simulink model "main"  (R2022a)
settings: Solver=ode3  StartTime=0.0  StopTime=10.0  RelTol=1e-3  EnableMultiTasking=on
model workspace (MAT data in the model file):
  BER = 1e-09
  Br = 1000000000
  Dr = 0.01
  Dt = 0.01
  F = 6
  G = 200
  GT = 0.012
  Ib = 5e-10
  Id = 1e-09
  Is = 5e-09
  Keff = 0.01
  Lil = -2
  Lin = -1.5
  Lout = -1.5
  M = 4
  Mer = 12
  Pavg = 0.0065
  Pback = 1e-13
  Pmax = 0.012
  Pmin = 0.001
  RIN = -145
  Rl = 100
  Tr = 300
  d = 1000
  d_gamma = 1e-09
  ja = 1e-05
  k = 2
  lambda = 8.5e-07
  n = 0.59
  nr = 0.8
  nsp = 2
  nt = 0.8
  u = 1
settings Model: Creator=keged  LastModifiedBy=keged
settings SolverCC: AutoInsertRateTranBlk=on
settings DataIOCC: SaveOutput=off  SaveTime=off
settings OptimizationCC: DefaultParameterBehavior=Inlined  InlineInvariantSignals=on  EnhancedBackFolding=on  PassReuseOutputArgsAs=Individual arguments  StateBitsets=on  DataBitsets=on  ZeroExternalMemoryAtStartup=off  ZeroInternalMemoryAtStartup=off  NoFixptDivByZeroProtection=on  LifeSpan=1  OptimizeBlockOrder=speed  DifferentSizesBufferReuse=on  EfficientTunableParamExpr=on
settings DebuggingCC: ParameterTunabilityLossMsg=error
settings HardwareCC: ProdBitPerPointer=32  ProdBitPerSizeT=32  ProdBitPerPtrDiffT=32  ProdLargestAtomicFloat=None  ProdIntDivRoundTo=Floor  ProdWordSize=32  ProdHWDeviceType=Generic->Custom
settings SFSimCC: MATLABDynamicMemAlloc=off
settings RTWCC: SystemTargetFile=ert.tlc  TLCOptions=-p0  GenCodeOnly=on  TemplateMakefile=ert_default_tmf  GenerateReport=on  RTWVerbose=off  IncludeHyperlinkInReport=on  LaunchReport=on
settings CodeAppCC: ForceParamTrailComments=on  IgnoreCustomStorageClasses=off  OperatorAnnotations=on  SimulinkDataObjDesc=on  SFDataObjDesc=on  CustomSymbolStrGlobalVar=rt$N$M  CustomSymbolStrType=$N$M  CustomSymbolStrFcn=$N$M$F  CustomSymbolStrMacro=$N$M  InsertBlockDesc=on
settings ERTTargetCC: TargetLangStandard=C99 (ISO)  CodeReplacementLibrary=ISO_C  GenerateSampleERTMain=on  IncludeMdlTerminateFcn=off  SuppressErrorStatus=on  SupportAbsoluteTime=off  PurelyIntegerCode=on  SupportNonFinite=off  SupportComplex=off  InlinedParameterPlacement=NonHierarchical  RootIOFormat=Structure reference  ERTCustomFileTemplate=example_file_process.tlc

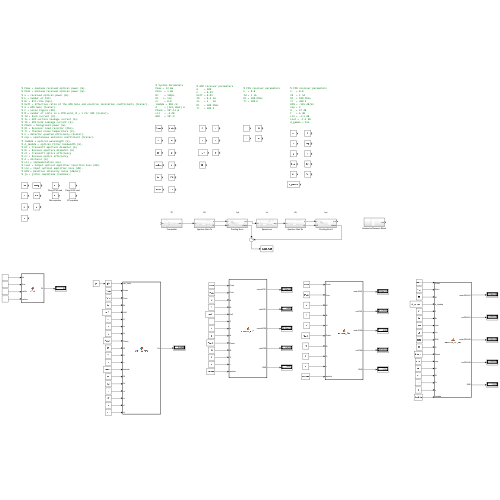
[thumbnail: Simulink's stored preview of the top-level diagram]
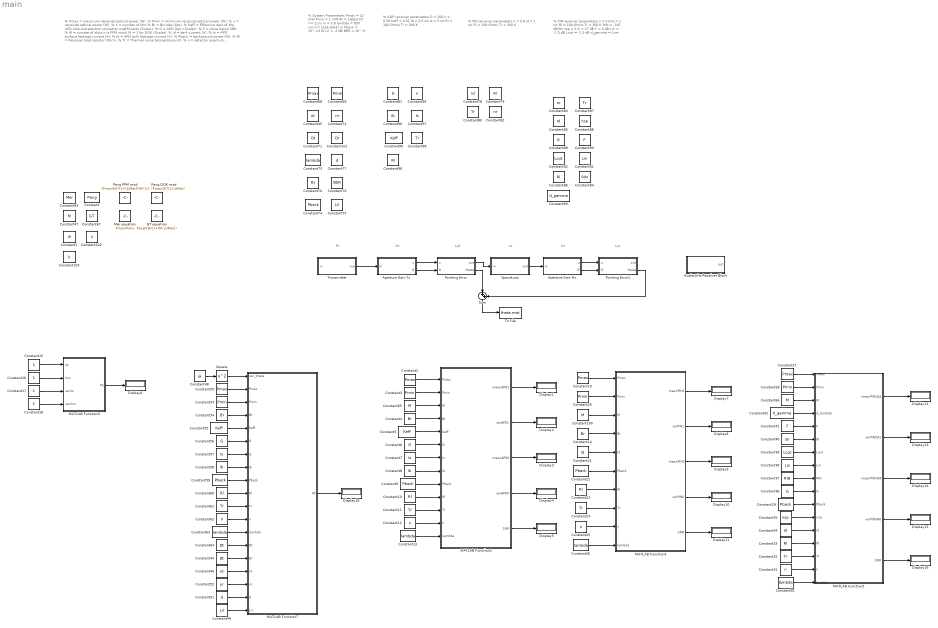
== system main ==
  note: Pt
  note: % PIN receiver parameters
      | n = 0.8
      | Id = 1 nA
      | Rl = 100 Ohms
      | Tr = 300 K
  note: % Pmax = maximum received optical power (W).
      | % Pmin = minimum received optical power (W).
      | % u = received optical power (W).
      | % k = number of bits
      | % Br = Bit rate (bps).
      | % Keff = Effective ratio of the APD hole and electron ionization coefficients (Scalar).
      | % G = APD Gain (Scalar).
      | % F = noise figure (dB).
      | % M = number of slots in a PPM word, M = 1 for OOK (Scalar).
      | % Id = dark current (A).
      | % Is = APD surface leakage current (A).
      | % Ib = APD bulk leakage current (A).
      | % Pback = background power (W).
      | % Rl = Receiver load resistor (Ohm).
      | % Tr = Thermal noise temperature (K).
      | % n = detector quantum efficiency (Scalar).
      | % nsp = spontaneous emission coefficient (Scalar).
      | % lambda = optical wavelength (m).
      | % d_lambda = optical filter bandwidth (m).
      | % Dt = Transmitt aperture diameter (m)
      | % Dr = Recieve aperture diameter (m)
      | % nt = Transmitt optics efficiency
      | % nr = Recieve optics efficiency
      | % d = distance (m)
      | % Lil = implementation loss
      | % Lout = Output optical amplifier insertion loss (dB).
      | % Lin = Input optical amplifier loss (dB).
      | % RIN = Relative intensity noise (dB/Hz).
      | % ja = jitter amplitude (radians).
  note: % ADP receiver parameters
      | G = 200
      | n = 0.59
      | Keff = 0.01
      | Ib = 0.5 nA
      | Is = 5 nA
      | Rl = 100 Ohms
      | Tr = 300 K
  note: % PIN receiver parameters
      | n = 0.8
      | Id = 1 nA
      | Rl = 100 Ohms
      | Tr = 300 K
      | RIN = -145 dB/Hz
      | nsp = 2
      | G = 27 dB
      | F = 6 dB
      | Lin = -1.5 dB
      | Lout = -1.5 dB
      | d_gamma = 1nm
  note: % System Parameters
      | Pmax = 12 mW
      | Pmin = 1 mW
      | Br = 1Gbps
      | Dt <= 1cm
      | nr = 0.8
      | lambda = 850 cm
      | d = [1e3,10e3] m
      | Pback = 10^-13 W
      | Lil = -2 dB
      | BER = 10^-9
  note: Gt
  note: Lpt
  note: Ls
  note: Lpr
  note: Gr
  Aperture Gain Rx : Subsystem
  Aperture Gain Tx : Subsystem
  Avalanche Receiver Block : Subsystem
  Constant : Constant  Value=Pavg
  Constant1 : Constant  Value=ja
  Constant{10,23,33,60,79,86,98} (7 alike) : Constant  Value=Rl
  Constant{47,65..66,100} (4 alike) : Constant  Value=M
  Constant101 : Constant  Value=Dr
  Constant102 : Constant  Value=u
  Constant103 : Constant  Value=k
  Constant{11,24,32,61,80,87,99} (7 alike) : Constant  Value=Tr
  Constant{12,25,31,62,94} (5 alike) : Constant  Value=n
  Constant{13,26,30,63,73} (5 alike) : Constant  Value=lambda
  Constant{4,14,40,54,70} (5 alike) : Constant  Value=Br
  Constant{15..18} (4 alike) : Constant
  Constant{2,19,27,50,68} (5 alike) : Constant  Value=Pmax
  Constant{3,20,28,53,69} (5 alike) : Constant  Value=Pmin
  Constant{21,34,78,85} (4 alike) : Constant  Value=Id
  Constant{9,22,29,59,74} (5 alike) : Constant  Value=Pback
  Constant35 : Constant  Value=nsp
  Constant{6,36,56,81,89} (5 alike) : Constant  Value=G
  Constant37 : Constant  Value=RIN
  Constant38 : Constant  Value=Lin
  Constant39 : Constant  Value=Lout
  Constant41 : Constant  Value=F
  Constant42 : Constant  Value=d_gamma
  Constant43 : Constant  Value=Mer
  Constant44 : Constant  Value=Dt
  Constant45 : Constant  Value=nt
  Constant46 : Constant  Value=nt
  Constant48 : Constant  Value=ja
  Constant49 : Constant  Value=Lil
  Constant5 : Constant  Value=Keff
  Constant51 : Constant  Value=d
  Constant{52,72,82..83} (4 alike) : Constant  Value=nr
  Constant55 : Constant  Value=Keff
  Constant57 : Constant  Value=Is
  Constant58 : Constant  Value=Ib
  Constant64 : Constant  Value=Dt
  Constant67 : Constant  Value=GT
  Constant7 : Constant  Value=Is
  Constant71 : Constant  Value=Dt
  Constant75 : Constant  Value=Lil
  Constant76 : Constant  Value=BER
  Constant77 : Constant  Value=d
  Constant8 : Constant  Value=Ib
  Constant84 : Constant  Value=RIN
  Constant88 : Constant  Value=nsp
  Constant90 : Constant  Value=F
  Constant91 : Constant  Value=Lin
  Constant92 : Constant  Value=Lout
  Constant93 : Constant  Value=d_gamma
  Constant95 : Constant  Value=Keff
  Constant96 : Constant  Value=Ib
  Constant97 : Constant  Value=Is
  Display{1..16,18} (17 alike) : Display
  GT equation : Constant  Value=Pavg*(M/(1+(M-1)/Mer))
  MATLAB Function2 : MATLAB Function  TreatAsAtomicUnit=on  RTWFcnName=Pointing
      settings: RTWFcnNameOpts=Use subsystem name  RTWFileNameOpts=Use subsystem name
  MATLAB Function3 : MATLAB Function  TreatAsAtomicUnit=on  RTWFcnName=Pointing
      settings: RTWFcnNameOpts=Use subsystem name  RTWFileNameOpts=Use subsystem name
  MATLAB Function4 : MATLAB Function  TreatAsAtomicUnit=on  RTWFcnName=Pointing
      settings: RTWFcnNameOpts=Use subsystem name  RTWFileNameOpts=Use subsystem name
  MATLAB Function5 : MATLAB Function  TreatAsAtomicUnit=on  RTWFcnName=Pointing
      settings: RTWFcnNameOpts=Use subsystem name  RTWFileNameOpts=Use subsystem name
  MATLAB Function7 : MATLAB Function  TreatAsAtomicUnit=on  RTWFcnName=Pointing
      settings: RTWFcnNameOpts=Use subsystem name  RTWFileNameOpts=Use subsystem name
  Mer equation : Constant  Value=Pmax/Pmin
  Pavg OOK mod : Constant  Value=(Pmax/2)*(1+1/Mer)
  Pavg PPM mod : Constant  Value=(Pmax/M)*(1+(1/Mer)*(M-1))
  Pointing Error : Subsystem
  Pointing Error1 : Subsystem
  SpaceLoss : Subsystem
  Square : Math  Operator=square
  Sum : Sum  Inputs=|++
  To File : ToFile  Filename=theta.mat  SaveFormat=Timeseries
  Transmitter : Subsystem
  wires:
  MATLAB Function2/1(meanAPD1) -> Display1/1
  Constant3/1 -> MATLAB Function2/2(Pmin)
  Constant2/1 -> MATLAB Function2/1(Pmax)
  Constant65/1 -> MATLAB Function2/3(M)
  Constant4/1 -> MATLAB Function2/4(Br)
  Constant5/1 -> MATLAB Function2/5(Keff)
  Constant6/1 -> MATLAB Function2/6(G)
  Constant7/1 -> MATLAB Function2/7(Is)
  Constant8/1 -> MATLAB Function2/8(Ib)
  Constant9/1 -> MATLAB Function2/9(Pback)
  Constant10/1 -> MATLAB Function2/10(Rl)
  Constant11/1 -> MATLAB Function2/11(Tr)
  Constant12/1 -> MATLAB Function2/12(n)
  Constant13/1 -> MATLAB Function2/13(lambda)
  MATLAB Function2/2(varAPD1) -> Display2/1
  MATLAB Function2/3(meanAPD0) -> Display3/1
  MATLAB Function2/4(varAPD0) -> Display4/1
  MATLAB Function2/5(SNR) -> Display5/1
  MATLAB Function3/1(Pb) -> Display6/1
  Constant16/1 -> MATLAB Function3/2(Xns)
  Constant15/1 -> MATLAB Function3/1(Xs)
  Constant17/1 -> MATLAB Function3/3(varXs)
  Constant18/1 -> MATLAB Function3/4(varXns)
  MATLAB Function4/4(varPIN0) -> Display10/1
  MATLAB Function4/5(SNR) -> Display11/1
  Constant100/1 -> MATLAB Function4/3(M)
  Constant24/1 -> MATLAB Function4/8(Tr)
  Constant22/1 -> MATLAB Function4/6(Pback)
  MATLAB Function4/2(varPIN1) -> Display8/1
  Constant21/1 -> MATLAB Function4/5(Id)
  MATLAB Function4/3(meanPIN0) -> Display9/1
  Constant23/1 -> MATLAB Function4/7(Rl)
  MATLAB Function4/1(meanPIN1) -> Display7/1
  Constant25/1 -> MATLAB Function4/9(n)
  Constant14/1 -> MATLAB Function4/4(Br)
  Constant20/1 -> MATLAB Function4/2(Pmin)
  Constant26/1 -> MATLAB Function4/10(lambda)
  Constant19/1 -> MATLAB Function4/1(Pmax)
  MATLAB Function5/4(varPINOA0) -> Display15/1
  MATLAB Function5/5(SNR) -> Display16/1
  Constant41/1 -> MATLAB Function5/5(F)
  Constant66/1 -> MATLAB Function5/3(M)
  Constant39/1 -> MATLAB Function5/7(Lout)
  Constant32/1 -> MATLAB Function5/15(Tr)
  Constant29/1 -> MATLAB Function5/11(Pback)
  MATLAB Function5/2(varPINOA1) -> Display13/1
  Constant36/1 -> MATLAB Function5/10(G)
  Constant42/1 -> MATLAB Function5/4(d_lambda)
  MATLAB Function5/3(meanPINOA0) -> Display14/1
  Constant33/1 -> MATLAB Function5/14(Rl)
  MATLAB Function5/1(meanPINOA1) -> Display12/1
  Constant31/1 -> MATLAB Function5/16(n)
  Constant40/1 -> MATLAB Function5/6(Br)
  Constant28/1 -> MATLAB Function5/2(Pmin)
  Constant30/1 -> MATLAB Function5/17(lambda)
  Constant27/1 -> MATLAB Function5/1(Pmax)
  Constant34/1 -> MATLAB Function5/13(Id)
  Constant35/1 -> MATLAB Function5/12(nsp)
  Constant37/1 -> MATLAB Function5/9(RIN)
  Constant38/1 -> MATLAB Function5/8(Lin)
  MATLAB Function7/1(Pb) -> Display18/1
  Square/1 -> MATLAB Function7/1(var_theta)
  Constant50/1 -> MATLAB Function7/2(Pmax)
  Constant53/1 -> MATLAB Function7/3(Pmin)
  Constant54/1 -> MATLAB Function7/4(Br)
  Constant55/1 -> MATLAB Function7/5(Keff)
  Constant56/1 -> MATLAB Function7/6(G)
  Constant57/1 -> MATLAB Function7/7(Is)
  Constant58/1 -> MATLAB Function7/8(Ib)
  Constant59/1 -> MATLAB Function7/9(Pback)
  Constant60/1 -> MATLAB Function7/10(Rl)
  Constant61/1 -> MATLAB Function7/11(Tr)
  Constant62/1 -> MATLAB Function7/12(n)
  Constant63/1 -> MATLAB Function7/13(lambda)
  Constant64/1 -> MATLAB Function7/14(Dt)
  Constant44/1 -> MATLAB Function7/15(Dr)
  Constant46/1 -> MATLAB Function7/16(nt)
  Constant52/1 -> MATLAB Function7/17(nr)
  Constant51/1 -> MATLAB Function7/18(d)
  Constant49/1 -> MATLAB Function7/19(Lil)
  Transmitter/1(out) -> Aperture Gain Tx/1(in)
  Aperture Gain Tx/1(u) -> Pointing Error/1(u)
  Aperture Gain Tx/2(G) -> Pointing Error/2(G)
  Constant48/1 -> Square/1
  Pointing Error/1(out) -> SpaceLoss/1(in)
  SpaceLoss/1(out) -> Aperture Gain Rx/1(in)
  Pointing Error/2(theta) -> Sum/1
  Sum/1 -> To File/1
  Aperture Gain Rx/1(u) -> Pointing Error1/1(u)
  Aperture Gain Rx/2(G) -> Pointing Error1/2(G)
  Pointing Error1/2(theta) -> Sum/2

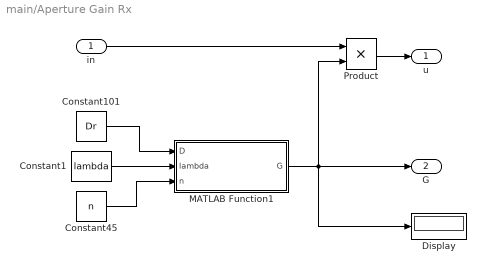
== system main/Aperture Gain Rx ==
  in : Inport
  Constant1 : Constant  Value=lambda
  Constant101 : Constant  Value=Dr
  Constant45 : Constant  Value=n
  Display : Display
  MATLAB Function1 : MATLAB Function  TreatAsAtomicUnit=on  RTWFcnName=Pointing
      settings: RTWFcnNameOpts=Use subsystem name  RTWFileNameOpts=Use subsystem name
  Product : Product
  u : Outport
  G : Outport  Port=2
  wires:
  Constant101/1 -> MATLAB Function1/1(D)
  Constant45/1 -> MATLAB Function1/3(n)
  Constant1/1 -> MATLAB Function1/2(lambda)
  MATLAB Function1/1(G) -> Display/1, Product/2, G/1
  Product/1 -> u/1
  in/1 -> Product/1

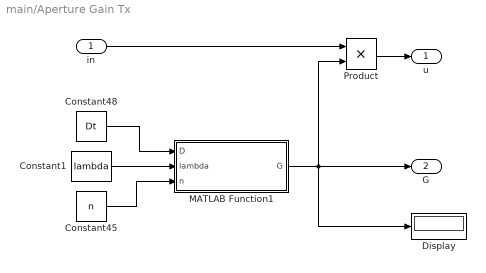
== system main/Aperture Gain Tx ==
  in : Inport
  Constant1 : Constant  Value=lambda
  Constant45 : Constant  Value=n
  Constant48 : Constant  Value=Dt
  Display : Display
  MATLAB Function1 : MATLAB Function  TreatAsAtomicUnit=on  RTWFcnName=Pointing
      settings: RTWFcnNameOpts=Use subsystem name  RTWFileNameOpts=Use subsystem name
  Product : Product
  u : Outport
  G : Outport  Port=2
  wires:
  Constant48/1 -> MATLAB Function1/1(D)
  Constant45/1 -> MATLAB Function1/3(n)
  Constant1/1 -> MATLAB Function1/2(lambda)
  MATLAB Function1/1(G) -> Display/1, Product/2, G/1
  Product/1 -> u/1
  in/1 -> Product/1

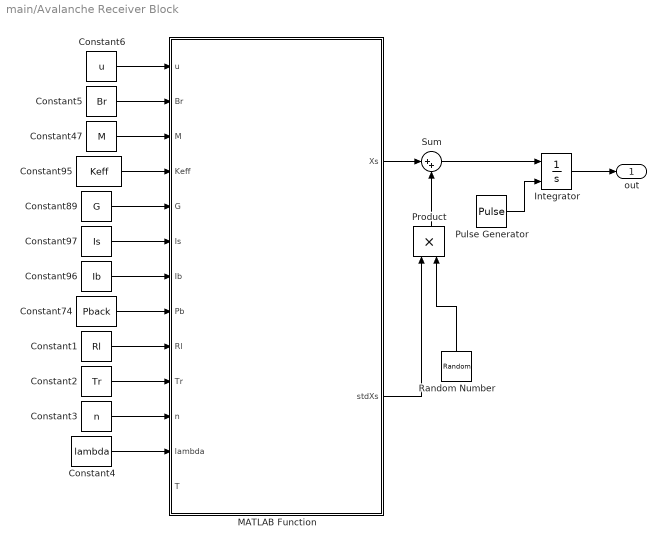
== system main/Avalanche Receiver Block ==
  Constant1 : Constant  Value=Rl
  Constant2 : Constant  Value=Tr
  Constant3 : Constant  Value=n
  Constant4 : Constant  Value=lambda
  Constant47 : Constant  Value=M
  Constant5 : Constant  Value=Br
  Constant6 : Constant  Value=u
  Constant74 : Constant  Value=Pback
  Constant89 : Constant  Value=G
  Constant95 : Constant  Value=Keff
  Constant96 : Constant  Value=Ib
  Constant97 : Constant  Value=Is
  Integrator : Integrator  ExternalReset=rising
  MATLAB Function : MATLAB Function  TreatAsAtomicUnit=on
  Product : Product
  Pulse Generator : DiscretePulseGenerator  PulseType=Time based  Period=k/Br  PulseWidth=k/M/Br
  Random Number : RandomNumber  SampleTime=0.1
  Sum : Sum  Inputs=|++
  out : Outport
  wires:
  Constant47/1 -> MATLAB Function/3(M)
  Constant95/1 -> MATLAB Function/4(Keff)
  Constant89/1 -> MATLAB Function/5(G)
  Constant97/1 -> MATLAB Function/6(Is)
  Constant96/1 -> MATLAB Function/7(Ib)
  Constant1/1 -> MATLAB Function/9(Rl)
  Constant2/1 -> MATLAB Function/10(Tr)
  Constant3/1 -> MATLAB Function/11(n)
  Constant4/1 -> MATLAB Function/12(lambda)
  Constant6/1 -> MATLAB Function/1(u)
  Constant5/1 -> MATLAB Function/2(Br)
  Constant74/1 -> MATLAB Function/8(Pb)
  MATLAB Function/2(stdXs) -> Product/1
  Random Number/1 -> Product/2
  Product/1 -> Sum/2
  MATLAB Function/1(Xs) -> Sum/1
  Integrator/1 -> out/1
  Sum/1 -> Integrator/1
  Pulse Generator/1 -> Integrator/2

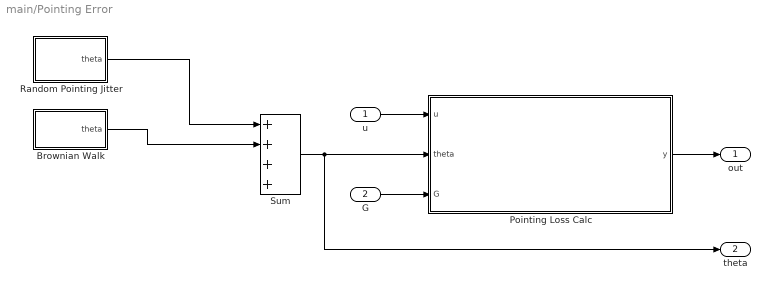
== system main/Pointing Error ==
  u : Inport
  G : Inport  Port=2
  Brownian Walk : Subsystem
  Pointing Loss Calc : Subsystem
  Random Pointing Jitter : Subsystem
  Sum : Sum  Inputs=++++  InputSameDT=on
  out : Outport
  theta : Outport  Port=2
  wires:
  u/1 -> Pointing Loss Calc/1(u)
  Pointing Loss Calc/1(y) -> out/1
  G/1 -> Pointing Loss Calc/3(G)
  Random Pointing Jitter/1(theta) -> Sum/1
  Sum/1 -> Pointing Loss Calc/2(theta), theta/1
  Brownian Walk/1(theta) -> Sum/2

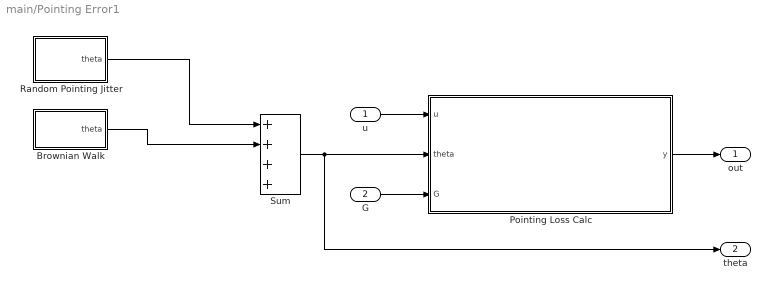
== system main/Pointing Error1 ==
  u : Inport
  G : Inport  Port=2
  Brownian Walk : Subsystem
  Pointing Loss Calc : Subsystem
  Random Pointing Jitter : Subsystem
  Sum : Sum  Inputs=++++  InputSameDT=on
  out : Outport
  theta : Outport  Port=2
  wires:
  u/1 -> Pointing Loss Calc/1(u)
  Pointing Loss Calc/1(y) -> out/1
  G/1 -> Pointing Loss Calc/3(G)
  Random Pointing Jitter/1(theta) -> Sum/1
  Sum/1 -> theta/1, Pointing Loss Calc/2(theta)
  Brownian Walk/1(theta) -> Sum/2

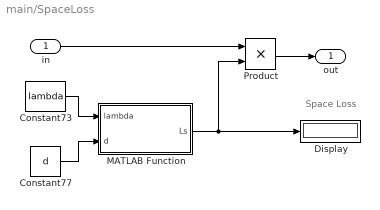
== system main/SpaceLoss ==
  note: Space Loss
  in : Inport
  Constant73 : Constant  Value=lambda
  Constant77 : Constant  Value=d
  Display : Display
  MATLAB Function : MATLAB Function  TreatAsAtomicUnit=on
  Product : Product
  out : Outport
  wires:
  MATLAB Function/1(Ls) -> Display/1, Product/2
  in/1 -> Product/1
  Product/1 -> out/1
  Constant73/1 -> MATLAB Function/1(lambda)
  Constant77/1 -> MATLAB Function/2(d)

== system main/Transmitter ==
  in : Inport
  Constant : Constant
  Constant1 : Constant  Value=1/Mer
  Gain : Gain  Gain=GT
  Switch : Switch  Criteria=u2 > Threshold  SaturateOnIntegerOverflow=off  InputSameDT=off
  out : Outport
  wires:
  in/1 -> Switch/2
  Constant/1 -> Switch/1
  Constant1/1 -> Switch/3
  Gain/1 -> out/1
  Switch/1 -> Gain/1

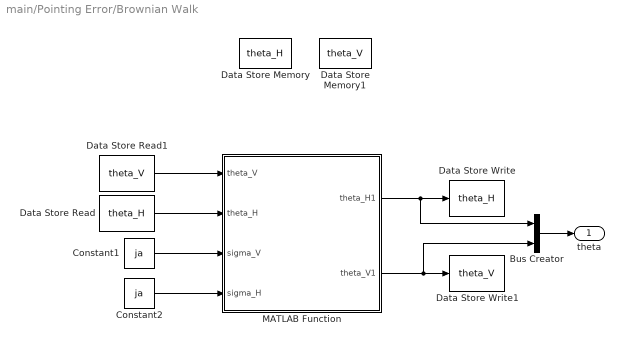
== system main/Pointing Error/Brownian Walk ==
  Bus Creator : BusCreator  Inputs=2
  Constant1 : Constant  Value=ja
  Constant2 : Constant  Value=ja
  Data Store Memory : DataStoreMemory  DataStoreName=theta_H  WriteAfterWriteMsg=warning  ShowAdditionalParam=off
  Data Store Memory1 : DataStoreMemory  DataStoreName=theta_V  WriteAfterWriteMsg=warning  ShowAdditionalParam=off
  Data Store Read : DataStoreRead  DataStoreName=theta_H  IndexOptions=Index vector (dialog)  Indices=1  OutputSizes=1
  Data Store Read1 : DataStoreRead  DataStoreName=theta_V  IndexOptions=Index vector (dialog)  Indices=1  OutputSizes=1
  Data Store Write : DataStoreWrite  DataStoreName=theta_H  IndexOptions=Index vector (dialog)  Indices=1  OutputSizes=1
  Data Store Write1 : DataStoreWrite  DataStoreName=theta_V  IndexOptions=Index vector (dialog)  Indices=1  OutputSizes=1
  MATLAB Function : MATLAB Function  TreatAsAtomicUnit=on
  theta : Outport
  wires:
  MATLAB Function/1(theta_H1) -> Bus Creator/1, Data Store Write/1
  Data Store Read/1 -> MATLAB Function/2(theta_H)
  Data Store Read1/1 -> MATLAB Function/1(theta_V)
  MATLAB Function/2(theta_V1) -> Bus Creator/2, Data Store Write1/1
  Bus Creator/1 -> theta/1
  Constant1/1 -> MATLAB Function/3(sigma_V)
  Constant2/1 -> MATLAB Function/4(sigma_H)

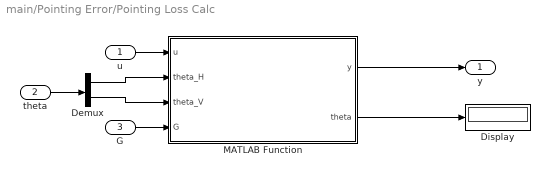
== system main/Pointing Error/Pointing Loss Calc ==
  u : Inport
  theta : Inport  Port=2
  G : Inport  Port=3
  Demux : Demux  Outputs=2
  Display : Display
  MATLAB Function : MATLAB Function  TreatAsAtomicUnit=on
  y : Outport
  wires:
  MATLAB Function/2(theta) -> Display/1
  G/1 -> MATLAB Function/4(G)
  u/1 -> MATLAB Function/1(u)
  MATLAB Function/1(y) -> y/1
  theta/1 -> Demux/1
  Demux/2 -> MATLAB Function/3(theta_V)
  Demux/1 -> MATLAB Function/2(theta_H)

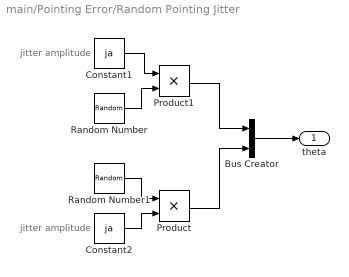
== system main/Pointing Error/Random Pointing Jitter ==
  note: jitter amplitude
  note: jitter amplitude
  Bus Creator : BusCreator  Inputs=2
  Constant1 : Constant  Value=ja
  Constant2 : Constant  Value=ja
  Product : Product
  Product1 : Product
  Random Number : RandomNumber  SampleTime=0.1
  Random Number1 : RandomNumber  SampleTime=0.1
  theta : Outport
  wires:
  Random Number1/1 -> Product/1
  Constant2/1 -> Product/2
  Constant1/1 -> Product1/1
  Random Number/1 -> Product1/2
  Product1/1 -> Bus Creator/1
  Product/1 -> Bus Creator/2
  Bus Creator/1 -> theta/1

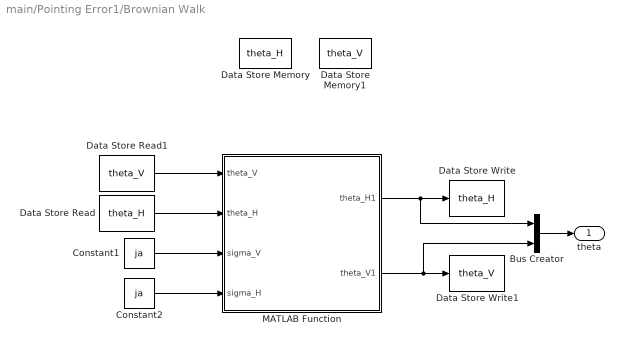
== system main/Pointing Error1/Brownian Walk ==
  Bus Creator : BusCreator  Inputs=2
  Constant1 : Constant  Value=ja
  Constant2 : Constant  Value=ja
  Data Store Memory : DataStoreMemory  DataStoreName=theta_H  WriteAfterWriteMsg=warning  ShowAdditionalParam=off
  Data Store Memory1 : DataStoreMemory  DataStoreName=theta_V  WriteAfterWriteMsg=warning  ShowAdditionalParam=off
  Data Store Read : DataStoreRead  DataStoreName=theta_H  IndexOptions=Index vector (dialog)  Indices=1  OutputSizes=1
  Data Store Read1 : DataStoreRead  DataStoreName=theta_V  IndexOptions=Index vector (dialog)  Indices=1  OutputSizes=1
  Data Store Write : DataStoreWrite  DataStoreName=theta_H  IndexOptions=Index vector (dialog)  Indices=1  OutputSizes=1
  Data Store Write1 : DataStoreWrite  DataStoreName=theta_V  IndexOptions=Index vector (dialog)  Indices=1  OutputSizes=1
  MATLAB Function : MATLAB Function  TreatAsAtomicUnit=on
  theta : Outport
  wires:
  MATLAB Function/1(theta_H1) -> Bus Creator/1, Data Store Write/1
  Data Store Read/1 -> MATLAB Function/2(theta_H)
  Data Store Read1/1 -> MATLAB Function/1(theta_V)
  MATLAB Function/2(theta_V1) -> Bus Creator/2, Data Store Write1/1
  Bus Creator/1 -> theta/1
  Constant1/1 -> MATLAB Function/3(sigma_V)
  Constant2/1 -> MATLAB Function/4(sigma_H)

== system main/Pointing Error1/Pointing Loss Calc ==
  u : Inport
  theta : Inport  Port=2
  G : Inport  Port=3
  Demux : Demux  Outputs=2
  Display : Display
  MATLAB Function : MATLAB Function  TreatAsAtomicUnit=on
  y : Outport
  wires:
  MATLAB Function/2(theta) -> Display/1
  G/1 -> MATLAB Function/4(G)
  u/1 -> MATLAB Function/1(u)
  MATLAB Function/1(y) -> y/1
  theta/1 -> Demux/1
  Demux/1 -> MATLAB Function/2(theta_H)
  Demux/2 -> MATLAB Function/3(theta_V)

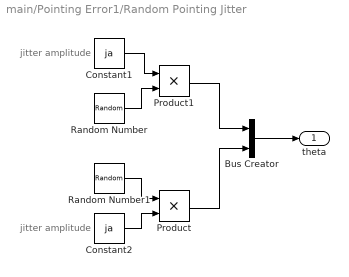
== system main/Pointing Error1/Random Pointing Jitter ==
  note: jitter amplitude
  note: jitter amplitude
  Bus Creator : BusCreator  Inputs=2
  Constant1 : Constant  Value=ja
  Constant2 : Constant  Value=ja
  Product : Product
  Product1 : Product
  Random Number : RandomNumber  SampleTime=0.1
  Random Number1 : RandomNumber  SampleTime=0.1
  theta : Outport
  wires:
  Random Number1/1 -> Product/1
  Constant2/1 -> Product/2
  Constant1/1 -> Product1/1
  Random Number/1 -> Product1/2
  Product1/1 -> Bus Creator/1
  Product/1 -> Bus Creator/2
  Bus Creator/1 -> theta/1

== matlab function main/Pointing Error/Brownian Walk/MATLAB Function ==
  data: theta_V input; theta_H1 output; theta_H input; sigma_V input; sigma_H input; theta_V1 output
function [theta_H1, theta_V1] = brownian_vib(theta_V, theta_H, sigma_V, sigma_H)

%Generates a stochastic random walking motion.
%Sets the standard deviation of the step size for the brownian walk.
d_sigma_H = sigma_H/100;

%Generates a step of random length and direction along the azimuthal axis.
d_theta_H = randn()*d_sigma_H - theta_H*d_sigma_H/sigma_H;

%the new error angle is produced by adding the random step the the current
%error angle.
theta_H1 = theta_H + d_theta_H;

%The same principle for the elevation axis.
d_sigma_V = sigma_V/100;
d_theta_V = randn()*d_sigma_V - theta_V*d_sigma_V/sigma_V;

theta_V1 = theta_V + d_theta_V;

end

== matlab function main/MATLAB Function7 ==
  data: var_theta input; Pmax input; Pb output; Pmin input; Br input; Keff input; G input; Is input; Ib input; Pback input; Rl input; Tr input; n input; lambda input; Dt input; Dr input; nt input; nr input; d input; Lil input
function Pb = OOK_vib_APD(var_theta, Pmax, Pmin, Br, Keff, G, Is, Ib,...
Pback, Rl, Tr, n, lambda, Dt, Dr, nt, nr, d, Lil)

% Solves the double integral that evaluates the mean BER for a certain
% standard deviation of the pointing jitter.
Pb = 0;
for theta_r = 0:2*10^-6:10^-4
	P = 0;
	for theta_t = 0:2*10^-6:10^-4
		P = P + P_OOK_theta(Pmax, Pmin, Br, Keff, G, Is, Ib, Pback, Rl,...
		Tr, n, lambda, theta_t, theta_r, Dt, Dr, nt, nr, d, Lil)*...
		raylpdf(theta_t, var_theta)*(2*10^-6);
	end
	Pb = Pb + P*raylpdf(theta_r, var_theta)*(2*10^-6);
end

end

%Gives the BER for a certain transmitter and receiver pointing error.

% Pmax = maximum received optical power (W).
% Pmin = minimum received optical power (W).
% Br = Bit rate (bps).
% Keff = Effective ratio of the APD hole and electron ionization
%        coefficients (Scalar).
% G = APD Gain (Scalar).
% Is = APD surface leakage current (A).
% Ib = APD bulk leakage current (A).
% Pback = incident background power (W).
% Rl = Receiver load resistor (Ohm).
% Tr = Thermal noise temperature (K).
% n = detector quantum efficiency (Scalar).
% lambda = optical wavelength (m).
% Dt = Transmitt aperture diameter (m)
% Dr = Recieve aperture diameter (m)
% nt = Transmitt optics efficiency
% nr = Recieve optics efficiency
% d = distance (m)
% Lil = implementation loss

function P_OOK = P_OOK_theta(Pmax, Pmin, Br, Keff, G, Is, Ib, Pback, Rl,...
Tr, n, lambda, theta_t, theta_r, Dt, Dr, nt, nr, d, Lil)

Pr1 = Pmax*PointingLoss(Ap_G(Dt, lambda, nt), theta_t)*Ap_G(Dt,lambda,nt)...
    *SpaceLoss(lambda,d)*PointingLoss(Ap_G(Dr, lambda, nr), theta_r)...
    *Ap_G(Dr,lambda,nr)*10^(-Lil/10);

Pr0 = Pmin*PointingLoss(Ap_G(Dt, lambda, nt), theta_t)*Ap_G(Dt,lambda,nt)...
    *SpaceLoss(lambda,d)*PointingLoss(Ap_G(Dr, lambda, nr), theta_r)...
    *Ap_G(Dr,lambda,nr)*10^(-Lil/10);

[Xs, varXs, Xns, varXns, SNR] = ...
meanvar_APD(Pr1, Pr0, 1, Br, Keff, G, Is, Ib, Pback, Rl, Tr, n, lambda);

P_OOK = OOK(Xs, Xns, varXs, varXns);

end

== matlab function main/Aperture Gain Tx/MATLAB Function1 ==
  data: D input; G output; lambda input; n input
function G = Ap_G(D, lambda, n)

% G = aperture gain
% D = aperture diameter (m)
% lambda = wavelength (m)
% n = optics efficiency
G=(pi*D/lambda)^2*n;

end

== matlab function main/SpaceLoss/MATLAB Function ==
  data: lambda input; Ls output; d input
function Ls = SpaceLoss(lambda, d)

% Ls = free-space loss
% lambda = wavelength (m)
% d = distance (m)
Ls = (lambda/(4*pi*d))^2;

end

== matlab function main/Aperture Gain Rx/MATLAB Function1 ==
  data: D input; G output; lambda input; n input
function G = Ap_G(D, lambda, n)

% G = aperture gain
% D = aperture diameter (m)
% lambda = wavelength (m)
% n = optics efficiency
G=(pi*D/lambda)^2*n;

end

== matlab function main/Pointing Error1/Brownian Walk/MATLAB Function ==
  data: theta_V input; theta_H1 output; theta_H input; sigma_V input; sigma_H input; theta_V1 output
function [theta_H1, theta_V1] = brownian_vib(theta_V, theta_H, sigma_V, sigma_H)

%Generates a stochastic random walking motion.
%Sets the standard deviation of the step size for the brownian walk.
d_sigma_H = sigma_H/100;

%Generates a step of random length and direction along the azimuthal axis.
d_theta_H = randn()*d_sigma_H - theta_H*d_sigma_H/sigma_H;

%the new error angle is produced by adding the random step the the current
%error angle.
theta_H1 = theta_H + d_theta_H;

%The same principle for the elevation axis.
d_sigma_V = sigma_V/100;
d_theta_V = randn()*d_sigma_V - theta_V*d_sigma_V/sigma_V;

theta_V1 = theta_V + d_theta_V;

end

== matlab function main/Pointing Error1/Pointing Loss Calc/MATLAB Function ==
  data: u input; y output; theta_H input; theta_V input; G input; theta output
function [y,theta] = PointingLossTheta(u, theta_H, theta_V, G)

% Calculates the "line of sight damping" between the transmitter and
% receiver due to the pointing error.

theta = sqrt(theta_V^2 + theta_H^2);
y = u*exp(-G*theta^2);

end

== matlab function main/Avalanche Receiver Block/MATLAB Function ==
  data: u input; Xs output; Br input; M input; Keff input; G input; Is input; Ib input; Pb input; Rl input; Tr input; n input; lambda input; stdXs output; T input
function [Xs, stdXs]=noise_ADP(u, Br, M, Keff, G, Is, Ib, Pb, Rl, Tr, n, lambda, T)

%u = Received optical power (W).
%Br = Bit rate (bps).
%M = The M number of the PPM (Scalar).
%Keff = Effective ratio of the APD hole and electron ionization
%coefficients (Scalar).
%G = APD Gain (Scalar).
%Is = APD surface leakage current (A).
%Ib = APD bulk leakage current (A).
%Pb = incident background power (W).
%Rl = Receiver load resistor (Ohm).
%Tr = Thermal noise temperature (K).
%n = detector quantum efficiency (Scalar).
%lambda = optical wavelength (m).
%T = period / pulse duration

q = 1.60217646*10^-19; % Electron charge (C).
Kb = 1.38065*10^-23; % Boltzmann (J/K).
h = 6.6260688*10^-34; % Plank (Js).
c = 299792458; % speed of light in vaccum (m/s).

f = c/lambda; % Optical frequency (Hz).
R = G*q*n/(h*f); % Responsivity of the APD (A/W).
Bw = Br*M/log2(M); % Occupied bandwidth of the modulation (Hz).
F = Keff*G + (1 - Keff)*(2 - 1/G); % APD excess noise figure (Scalar).

%The variances of different noise sources for an APD receiver.
varSn = 2*q*F*u*R*G*Bw; %Signal shot noise (A^2).
varDc = 2*q*F*G^2*Ib*Bw + 2*q*Bw*Is; %Dark current noise (A^2).
varBg = 2*q*F*Pb*R*G*Bw; %Background noise (A^2).
varTh = 4*Kb*Tr*Bw/Rl; %Thermal noise (A^2).

% Mean (A) and variance (A^2) for the input signal.
Xs = (R*u + R*Pb + G*Ib + Is)*T;

stdXs = sqrt((varSn + varBg + varDc + varTh)*T);

end

== matlab function main/Pointing Error/Pointing Loss Calc/MATLAB Function ==
  data: u input; y output; theta_H input; theta_V input; G input; theta output
function [y,theta] = PointingLossTheta(u, theta_H, theta_V, G)

% Calculates the "line of sight damping" between the transmitter and
% receiver due to the pointing error.

theta = sqrt(theta_V^2 + theta_H^2);
y = u*exp(-G*theta^2);

end

== matlab function main/MATLAB Function2 ==
  data: Pmax input; meanAPD1 output; Pmin input; M input; Br input; Keff input; G input; Is input; Ib input; Pback input; Rl input; Tr input; n input; lambda input; varAPD1 output; meanAPD0 output; varAPD0 output; SNR output
function [meanAPD1, varAPD1, meanAPD0, varAPD0, SNR] =...
meanvar_APD(Pmax, Pmin, M, Br, Keff, G, Is, Ib, Pback, Rl, Tr, n, lambda)

% Pmax = maximum received optical power (W).
% Pmin = minimum received optical power (W).
% M = Numder of slots in PPM, M = 1 for OOK (Scalar).
% Br = Bit rate (bps).
% Keff = Effective ratio of the APD hole and electron ionization
%        coefficients (Scalar).
% G = APD Gain (Scalar).
% Is = APD surface leakage current (A).
% Ib = APD bulk leakage current (A).
% Pback = incident background power (W).
% Rl = Receiver load resistor (Ohm).
% Tr = Thermal noise temperature (K).
% n = detector quantum efficiency (Scalar).
% lambda = optical wavelength (m).

q = 1.60217646*10^-19; % electron charge (C).
Kb = 1.38065*10^-23; % Boltzmann (J/K).
h = 6.6260688*10^-34; % plank (Js).
c = 299792458; % speed of light in vaccum (m/s).
f = c/lambda; % Optical frequency (Hz).
R = G*q*n/(h*f); % Responsivity of the APD (A/W).
Bw = Br*M/log2(M); % Occupied bandwidth of the modulation (Hz).

if M == 1 % Makes sure that OOK gets correct average power and bandwidth.
	Bw = Br;
	M = 2;
end

Pavg = Pmax*(1 + Pmin/Pmax*(M-1))/M; % Average received power (W).
F = Keff*G + (1 - Keff)*(2 - 1/G); % APD excess noise figure (Scalar).

%The variances of different noise sources for an APD receiver
varSn0 = 2*q*F*Pmin*R*G*Bw; %signal shot noise for "0" (A^2).
varSn1 = 2*q*F*Pmax*R*G*Bw; %signal shot noise for "1" (A^2).
varSnavg= 2*q*F*Pavg*R*G*Bw; %signal shot noise for average power (A^2).
varDc = 2*q*F*G^2*Ib*Bw + 2*q*Bw*Is; %Dark current noise (A^2).
varBg = 2*q*F*Pback*R*G*Bw; %background noise (A^2).
varTh = 4*Kb*Tr*Bw/Rl; %Thermal noise (A^2).

% Mean (A) and variance (A^2) for a "zero" signal.
meanAPD0 = R*Pmin + R*Pback + G*Ib + Is;
varAPD0 = varSn0 + varBg + varDc + varTh;

% Mean (A) and variance (A^2) for a "one" signal.
meanAPD1 = R*Pmax + R*Pback + G*Ib + Is;
varAPD1 = varSn1 + varBg + varDc + varTh;

% The signal to noise ratio depends on the average received signal power.
varAPDavg = varSnavg + varBg + varDc + varTh;
SNR = 10*log((R*Pavg)^2/(varAPDavg)); %dB

end

== matlab function main/MATLAB Function3 ==
  data: Xs input; Pb output; Xns input; varXs input; varXns input
function Pb = OOK(Xs, Xns, varXs, varXns)

% "normalized distance" between the threshold and the distribution mean
DN = (Xs - Xns)/(sqrt(varXs) + sqrt(varXns));

% Bit error probability
Pb = 1/2*erfc(DN/sqrt(2));

end

== matlab function main/MATLAB Function4 ==
  data: Pmax input; meanPIN1 output; Pmin input; M input; Br input; Id input; Pback input; Rl input; Tr input; n input; lambda input; varPIN1 output; meanPIN0 output; varPIN0 output; SNR output
function [meanPIN1, varPIN1, meanPIN0, varPIN0, SNR] =...
    meanvar_PIN(Pmax, Pmin, M, Br, Id, Pback, Rl, Tr, n, lambda)

% Pmax = received power for a "one" (W).
% Pmin = received power for a "zero" (W).
% M = number of slots in a PPM symbol, for the case of
% OOK modulation, M = 1 (Scalar).
% Br = Bit rate (bps).
% Id = dark current (A)
% Pback = received background optical power (W).
% Rl = Load resistance (ohm).
% Tr = thermal temperature (K).
% n = quantum efficiency (Scalar).
% lambda = optical wavelength (m).

q = 1.60217646*10^-19; % electron charge (C).
Kb = 1.38065*10^-23; % Boltzmann (J/K).
h = 6.6260688*10^-34; % plank (Js).
c = 299792458; % speed of light in vaccum (m/s).
f = c/lambda; % Optical frequency (Hz).
R = q*n/(h*f); % Responsivity of the PIN (A/W).
Bw = Br*M/log2(M); % Occupied bandwidth of the modulation (Hz).

if M == 1 % Makes sure that OOK gets correct average power and bandwidth.
    Bw = Br;
    M = 2;
end

Pavg = Pmax*(1 + Pmin/Pmax*(M-1))/M; % Average received power (W).

%The variances of different noise sources for a PIN receiver without
%optical amplifier.
varSn0 = 2*q*R*Pmin*Bw; %signal shot noise for "0" (A^2).
varSn1 = 2*q*R*Pmax*Bw; %signal shot noise for "1" (A^2).
varSnavg= 2*q*R*Pavg*Bw; %signal shot noise for average power (A^2).
varDc = 2*q*Id*Bw; %Dark current noise (A^2).
varBg = 2*q*Pback*R*Bw; %background noise (A^2).
varTh = 4*Kb*Tr*Bw/Rl; %Thermal noise (A^2).

% Mean (A) and variance (A^2) for a "zero" signal.
meanPIN0 = R*Pmin + R*Pback + Id;
varPIN0 = varSn0 + varBg + varDc + varTh;

% Mean (A) and variance (A^2) for a "one" signal.
meanPIN1 = R*Pmax + R*Pback + Id;
varPIN1 = varSn1 + varBg + varDc + varTh;

% The signal to noise ratio depends on the average received signal power.
varPINavg = varSnavg + varBg + varDc + varTh;
SNR = 10*log((R*Pavg)^2/(varPINavg)); %dB

end

== matlab function main/MATLAB Function5 ==
  data: Pmax input; meanPINOA1 output; Pmin input; M input; d_lambda input; F input; Br input; Lout input; Lin input; RIN input; G input; Pback input; nsp input; Id input; Rl input; Tr input; n input; lambda input; varPINOA1 output; meanPINOA0 output; varPINOA0 output; SNR output
function [meanPINOA1, varPINOA1, meanPINOA0, varPINOA0, SNR] =...
meanvar_PIN_OA(Pmax, Pmin, M, d_lambda, F, Br, Lout, Lin, RIN,...
G, Pback, nsp, Id, Rl, Tr, n, lambda)

% Pmax = received maximum power (W).
% Pmin = received minimum power (W).
% M = number of slots in a PPM word, M = 1 for OOK (Scalar).
% delta_lambda = optical filter bandwidth (m).
% F = noise figure (dB).
% Br = Bit rate (bps).
% Lout = Output optical amplifier insertion loss (dB).
% Lin = Input optical amplifier loss (dB).
% RIN = Relative intensity noise (dB/Hz).
% G = Optical amplifier gain (Scalar).
% Pback = Received background power (W).
% nsp = spontaneous emission coefficient (Scalar).
% Id = dark current (A).
% Rl = Load resistance (Ohm).
% Tr = thermal temperature (K).
% n = quantum efficiency (Scalar).
% lambda = optical wavelength (m).

q = 1.60217646*10^-19; % electron charge (C).
Kb = 1.38065*10^-23; % Boltzmann (J/K).
h = 6.6260688*10^-34; % plank (Js).
c = 299792458; % speed of light in vaccum (m/s).
f = c/lambda; % Optical frequency (Hz).
R = q*n/(h*f); % Responsivity of the PIN (A/W).
Bop = d_lambda*c/lambda^2; % Bop = optical filter bandwidth in the
% frequency domain (Hz).
Bw = Br*M/log2(M); % Occupied bandwidth of the modulation (Hz).

if M == 1 % Makes sure that OOK gets correct average power and bandwidth.
    Bw = Br;
    M = 2;
end

Pavg = Pmax*(1 + Pmin/Pmax*(M-1))/M; % Average received optical power (W).

%The variances of different noise sources.
%Amplified signal shot noise (A^2).
varSn_0 = 2*q*G*R*Pmin*Bw;
varSn_1 = 2*q*G*R*Pmax*Bw;
varSn_avg = 2*q*G*R*Pavg*Bw;

%Amplified source relative intensity noise (A^2).
varRIN_0 = 10^(RIN/10)*(R*G*Pmin)^2*Bw;
varRIN_1 = 10^(RIN/10)*(R*G*Pmax)^2*Bw;
varRIN_avg = 10^(RIN/10)*(R*G*Pavg)^2*Bw;

%Amplified signal-spontaneous beat noise (A^2).
varSgSp_0 = 4*R^2*Pmin*G*Lin*Lout^2*(G-1)*nsp*h*f*Bw;
varSgSp_1 = 4*R^2*Pmax*G*Lin*Lout^2*(G-1)*nsp*h*f*Bw;
varSgSp_avg = 4*R^2*Pavg*G*Lin*Lout^2*(G-1)*nsp*h*f*Bw;

%Dark current noise (A^2).
varDc = 2*q*Id*Bw;

%Thermal noise (A^2).
varTh = 4*Kb*Tr*F*Bw/Rl;

%Amplified background noise (A^2).
varBg = 2*q*G*R*Pback*Bw;

%Amplified spontaneous emissions (A^2).
varSe = 4*R*q*h*f*nsp*(G-1)*Lout^2*Bw*Bop;

%Amplified spontaneous-spontaneous beat noise (A^2).
varSpSp = 8*(R*Lout*(G-1)*nsp*h*f)^2*Bop*Bw;

%The mean (A) and variance (A^2) for the "1" signal.
meanPINOA1 = R*G*Pmax + R*Pback + Id;
varPINOA1 = varSn_1 + varRIN_1 + varSgSp_1 + varDc + varTh + varBg...
+ varSe + varSpSp;

%The mean (A) and variance (A^2) for the "0" signal.
meanPINOA0 = R*G*Pmin + R*Pback + Id;
varPINOA0 = varSn_0 + varRIN_0 + varSgSp_0 + varDc + varTh + varBg...
+ varSe + varSpSp;

%The signal to noise ratio depends on the average received signal power.
varPINOA_avg = varSn_avg + varRIN_avg + varSgSp_avg + varDc + varTh...
+ varBg + varSe + varSpSp;

SNR = 10*log((R*G*Pavg)^2/(varPINOA_avg)); %dB

end
